simulink model "IP_DLQ_EI"  (R2022b)
settings: Solver=VariableStepAuto  StartTime=0.0  StopTime=t_sim  RelTol=1e-3
undefined symbols (not defined in the file): b1, b2, deltaT, DiscIntNeverNeededParam, etag, etam, g, Kgi, KliftS_EuleroIndietro, km, kt, Lb, liftFun, Lp, mb, mp, Rm, xbar
settings Model: Creator=vince  LastModifiedBy=vince

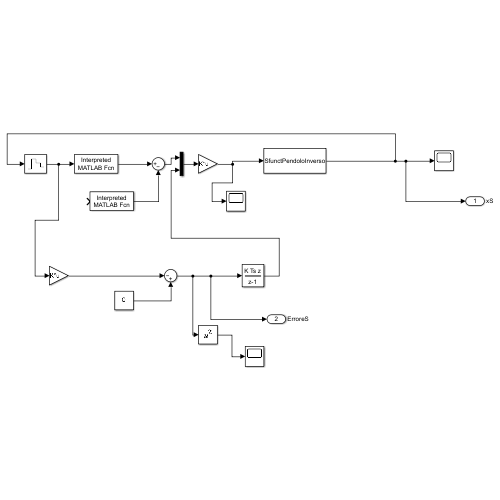
[thumbnail: Simulink's stored preview of the top-level diagram]
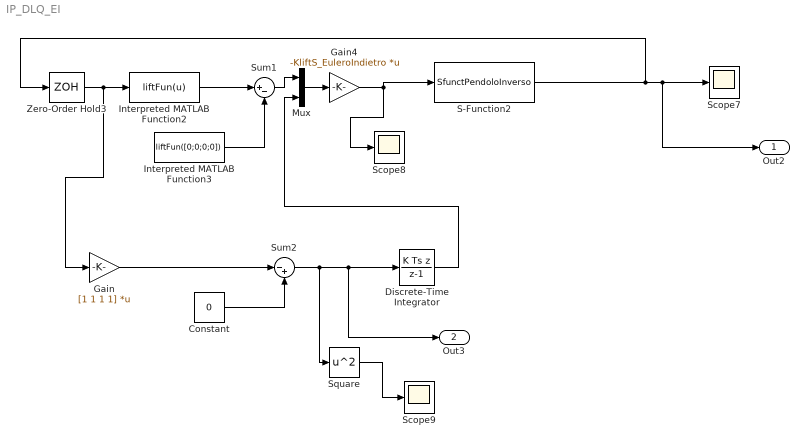
== system IP_DLQ_EI ==
  Constant : Constant  Value=0
  Discrete-Time Integrator : DiscreteIntegrator  IntegratorMethod=Integration: Backward Euler  SampleTime=deltaT  ICPrevOutput=DiscIntNeverNeededParam  ICPrevScaledInput=DiscIntNeverNeededParam
  Gain : Gain  Gain=[1 1 1 1]  Multiplication=Matrix(K*u)
  Gain4 : Gain  Gain=-KliftS_EuleroIndietro  Multiplication=Matrix(K*u)
  Interpreted MATLAB Function2 : MATLABFcn  MATLABFcn=liftFun(u)
  Interpreted MATLAB Function3 : MATLABFcn  MATLABFcn=liftFun([0;0;0;0])
  Mux : Mux  Inputs=2
  S-Function2 : S-Function  FunctionName=SfunctPendoloInverso  Parameters=xbar,mb,mp,Lb,Lp,b1,b2,g,Rm,kt,km,Kgi,etag,etam  SFunctionDeploymentMode=off  EnableBusSupport=off
  Scope7 : Scope
  Scope8 : Scope
  Scope9 : Scope
  Square : Math  Operator=square
  Sum1 : Sum  Inputs=|+-
  Sum2 : Sum  Inputs=|-+
  Zero-Order Hold3 : ZeroOrderHold  SampleTime=deltaT
  Out2 : Outport  SignalName=xS
  Out3 : Outport  Port=2  SignalName=ErroreS
  wires:
  Discrete-Time Integrator/1 -> Mux/2
  S-Function2/1 -> Out2/1, Scope7/1, Zero-Order Hold3/1
  Constant/1 -> Sum2/2
  Sum2/1 -> Square/1, Out3/1, Discrete-Time Integrator/1
  Square/1 -> Scope9/1
  Mux/1 -> Gain4/1
  Gain4/1 -> S-Function2/1, Scope8/1
  Interpreted MATLAB Function3/1 -> Sum1/2
  Zero-Order Hold3/1 -> Gain/1, Interpreted MATLAB Function2/1
  Sum1/1 -> Mux/1
  Gain/1 -> Sum2/1
  Interpreted MATLAB Function2/1 -> Sum1/1
